simulink model "Two_Level_SVM_No_PV_No_Control_Sw_Benchmark_v2"  (R2022b)
settings: Solver=FixedStepAuto  StartTime=0.0  StopTime=5  FixedStep=1e-7  RelTol=1e-3
model workspace (MAT data in the model file):
  Phase_Shift = Simulink.Parameter
  Phase_Shift.Value = 0.1974
  Phase_Shift.DataType = 'auto'
  Phase_Shift.Complexity = 'real'
  Phase_Shift.Dimensions = [1 1]
  Vrms_p = Simulink.Parameter
  Vrms_p.Value = 285.7229
  Vrms_p.DataType = 'auto'
  Vrms_p.Complexity = 'real'
  Vrms_p.Dimensions = [1 1]
libraries: spsIGBTDiodeLib x6, slpidlib x5, spsThreePhaseVIMeasurementLib x5, spsThreePhaseSeriesRLCBranchLib x4, spsGroundLib x2, spsabctodq0Lib x2, spsdq0toabcLib x1, spsDCVoltageSourceLib x1, spsThreePhaseProgrammableVoltageSourceLib x1, eeGeneralControl x1, spsabctoAlphaBetaZeroLib x1, eePwmGeneratorTwoLevel x1
(part 1 of 2)
settings Model: Creator=nitukeee  LastModifiedBy=buckb
settings OptimizationCC: LifeSpan=inf
settings DebuggingCC: SolverPrmCheckMsg=warning  UnconnectedInputMsg=warning  UnconnectedOutputMsg=warning  UnconnectedLineMsg=warning  SFUnexpectedBacktrackingDiag=warning  SFNoUnconditionalDefaultTransitionDiag=warning  SFExecutionAtInitializationDiag=none  SFMachineParentedDataDiag=warning  ArithmeticOperatorsInVariantConditions=warning
settings HardwareCC: ProdBitPerPointer=32  ProdBitPerSizeT=32  ProdBitPerPtrDiffT=32  ProdLargestAtomicFloat=None  ProdIntDivRoundTo=Undefined  ProdEndianess=Unspecified  ProdWordSize=32  ProdHWDeviceType=32-bit Generic
settings ModelReferenceCC: EnableRefExpFcnMdlSchedulingChecks=on  PropagateSignalLabelsOutOfModel=off
settings SFSimCC: SimUseLocalCustomCode=off  CustomCodeUndefinedFunction=UseInterfaceOnly
settings RTWCC: RTWUseLocalCustomCode=off  DLArmComputeVersion=19.05
settings CodeAppCC: StateflowObjectComments=on
settings GRTTargetCC: TargetLangStandard=C89/C90 (ANSI)
settings ConfigComp: CovMetricSettings=dw  CovSaveCumulativeToWorkspaceVar=on  CovSaveSingleToWorkspaceVar=on  CovExternalEMLEnable=off  CovSFcnEnable=off
settings SimscapeCC: SimscapeNormalizeSystem=off

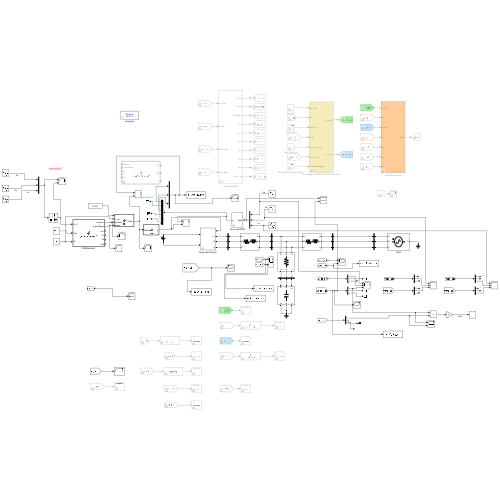
[thumbnail: Simulink's stored preview of the top-level diagram]
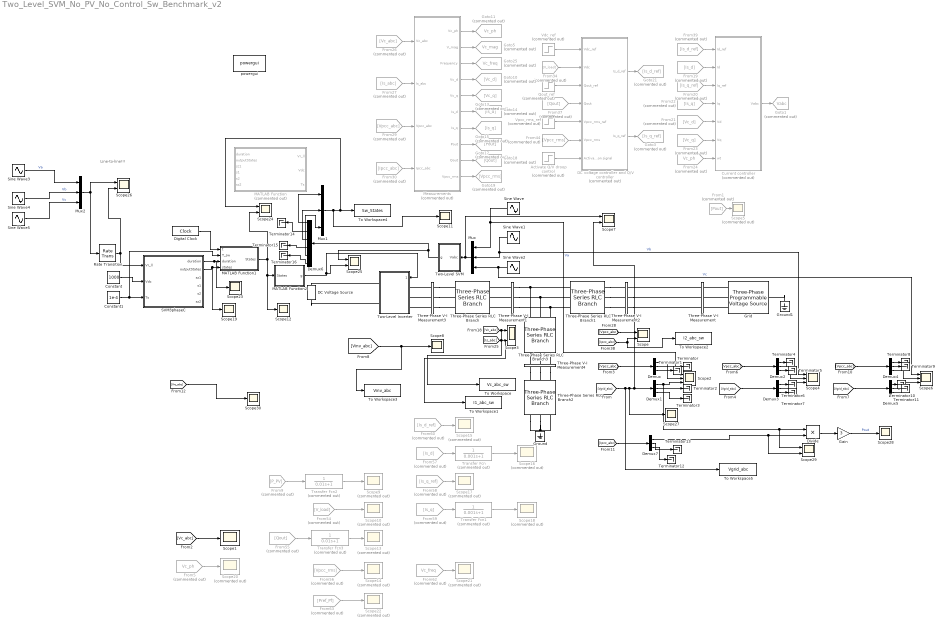
== system Two_Level_SVM_No_PV_No_Control_Sw_Benchmark_v2 ==
  note: Line-to-line!!!
  Activate Q/V droop control : Step  Commented=on  Time=3  After=0  SampleTime=0
  Constant : Constant  Value=1000
  Constant1 : Constant  Value=1e-4
  Current controller : Subsystem  Commented=on  mask{Kp_current_loop=0.59, Ki_current_loop=30, L1=3e-3, Udc_ref=1000, fsw=10e3}
      mask prompts: Kp_current_loop "Proportional parameter of current loop"; Ki_current_loop "Integral parameter of current loop"; L1 "Inverter-side inductor value [H]"; Udc_ref "DC voltage reference [V]"; fsw "Inverter switching frequency [Hz]"
      mask TypeOptions Kp_current_loop: Discrete PID Controller/P | Discrete PID Controller1/P
      mask TypeOptions Ki_current_loop: Discrete PID Controller/I | Discrete PID Controller1/I
      mask TypeOptions L1: L/Gain | L1/Gain
      mask TypeOptions Udc_ref: DC voltage/Value
      mask TypeOptions fsw:
      | PWM Generator
      | (Three-phase, Two-level)/fsw
  DC Voltage Source : spsDCVoltageSourceLib/DC Voltage Source  Amplitude=1000  Measurements=None
  DC voltage controller and Q/V controller : Subsystem  Commented=on  mask(DC voltage controller and Q/V controller){Kp_vdc_control=0.05, Ki_vdc_control=10, Kp_QV_control=1e-3, Ki_QV_control=1e-2, Dq=4.1667e+03}
      mask prompts: Kp_vdc_control "Proportional parameter of DC voltage controller"; Ki_vdc_control "Integratal parameter of DC voltage controller"; Kp_QV_control "Proportional parameter of Q/V controller"; Ki_QV_control "Integral parameter of Q/V controller"; Dq "Q/V droop constant [Var/V]"
      mask TypeOptions Kp_vdc_control: Discrete PID Controller/P
      mask TypeOptions Ki_vdc_control: Discrete PID Controller/I
      mask TypeOptions Kp_QV_control: Discrete PID Controller3/P
      mask TypeOptions Ki_QV_control: Discrete PID Controller3/I
      mask TypeOptions Dq: Dq/Gain
      mask DialogControl ParameterGroupVar1 Prompt: DC voltage controller
      mask DialogControl ParameterGroupVar2 Prompt: Q/V controller
  Demux{,1..5,7} (7 alike) : Demux  Outputs=3
  Demux6 : Demux  Outputs=6
  Digital Clock : DigitalClock  SampleTime=1e-7
  Divide : Product  Inputs=**
  From1 : From  Commented=on  GotoTag=Pout
  From19 : From  Commented=on  GotoTag=Is_d
  From20 : From  Commented=on  GotoTag=Is_q_ref
  From21 : From  Commented=on  GotoTag=Vc_d
  From22 : From  Commented=on  GotoTag=Is_q
  From23 : From  Commented=on  GotoTag=Vc_q
  From24 : From  Commented=on  GotoTag=Vc_ph  TagVisibility=global
  From26 : From  Commented=on  GotoTag=Vc_abc  TagVisibility=global
  From27 : From  Commented=on  GotoTag=Is_abc  TagVisibility=global
  From29 : From  Commented=on  GotoTag=Vpcc_abc  TagVisibility=global
  From30 : From  Commented=on  GotoTag=Ipcc_abc  TagVisibility=global
  From34 : From  Commented=on  GotoTag=V_load
  From37 : From  Commented=on  GotoTag=Qout
  From39 : From  Commented=on  GotoTag=Is_d_ref
  From44 : From  Commented=on  GotoTag=Vpcc_rms
  From5 : From  Commented=on  GotoTag=Vc_ph
  From54 : From  Commented=on  GotoTag=V_load
  From55 : From  Commented=on  GotoTag=Qout
  From56 : From  Commented=on  GotoTag=Vpcc_rms
  From57 : From  Commented=on  GotoTag=Is_d
  From58 : From  Commented=on  GotoTag=Is_q_ref
  From59 : From  Commented=on  GotoTag=Is_q
  From60 : From  Commented=on  GotoTag=Is_d_ref
  From62 : From  Commented=on  GotoTag=Vc_freq  TagVisibility=global
  From63 : From  Commented=on  GotoTag=Pref_Pf
  From9 : From  Commented=on  GotoTag=P_PV
  Gain : Gain  Gain=3
  Goto1 : Goto  Commented=on  GotoTag=Vabc  TagVisibility=global
  Goto10 : Goto  Commented=on  GotoTag=Vc_d
  Goto11 : Goto  Commented=on  GotoTag=Vc_ph  TagVisibility=global
  Goto13 : Goto  Commented=on  GotoTag=Vc_q
  Goto14 : Goto  Commented=on  GotoTag=Is_d
  Goto15 : Goto  Commented=on  GotoTag=Is_q
  Goto17 : Goto  Commented=on  GotoTag=Pout
  Goto18 : Goto  Commented=on  GotoTag=Qout
  Goto19 : Goto  Commented=on  GotoTag=Vpcc_rms
  Goto21 : Goto  Commented=on  GotoTag=Is_d_ref
  Goto25 : Goto  Commented=on  GotoTag=Vc_freq  TagVisibility=global
  Goto3 : Goto  Commented=on  GotoTag=Is_q_ref
  Goto5 : Goto  Commented=on  GotoTag=Vc_mag  TagVisibility=global
  Grid : spsThreePhaseProgrammableVoltageSourceLib/Three-Phase Programmable Voltage Source  PositiveSequence="[480  0 60]"  VariationEntity=None  VariationType=Table of time-amplitude pairs  VariationTypeAlt=Step  VariationStep=-0.1  VariationRate=10  VariationMagnitude=0.3  VariationFrequency=2  VariationTiming=[5.5 6.5]  VariationPhaseA=off  Amplitudes=[1 0.96 1.02]  TimeValues=[0 7 8.5]  HarmonicGeneration=off  HarmonicA=[3 0.2 -25 0]  HarmonicB=[2 0.15 35 2]  Timing="[0.05  3]"  BusType=swing  Pref=0  Qref=0  Qmin=-inf  Qmax=inf
  Ground : spsGroundLib/Ground  LConnTagsString=a
  Ground1 : spsGroundLib/Ground  LConnTagsString=a
  MATLAB Function : MATLAB Function  Commented=on  TreatAsAtomicUnit=on
  MATLAB Function1 : MATLAB Function  TreatAsAtomicUnit=on
  MATLAB Function2 : MATLAB Function  TreatAsAtomicUnit=on
  Measurements : Subsystem  Commented=on  mask{Kp_PLL=100, Ki_PLL=1e5}
      mask prompts: Kp_PLL "Proportional parameter of PLL"; Ki_PLL "Integral parameter of PLL"
      mask TypeOptions Kp_PLL: Phase Locked Loop (PLL)/Discrete PID Controller/P
      mask TypeOptions Ki_PLL: Phase Locked Loop (PLL)/Discrete PID Controller/I
  Mux : Mux  Inputs=3
  Mux1 : Mux  Inputs=3
  Mux2 : Mux  Inputs=3
  Qout_ref : Step  Commented=on  Time=0  After=0  SampleTime=0
  Rate Transition : RateTransition  OutPortSampleTime=1e-4
  SVM3phaseC : MATLAB Function  TreatAsAtomicUnit=on
  Scope{,3,7,24..26,29} (7 alike) : Scope  NumInputPorts=2
  Scope{1,8,11..12,19,23,27..28,30} (9 alike) : Scope
  Scope{5,9..10,13..18,20..22} (12 alike) : Scope  Commented=on
  Scope2 : Scope  NumInputPorts=3
  Scope4 : Scope  NumInputPorts=3
  Scope6 : Scope  NumInputPorts=3
  Sine Wave : Sin  Amplitude=Vrms_p*sqrt(2)  Frequency=2*pi*60  Phase=Phase_Shift  SampleTime=0
  Sine Wave1 : Sin  Amplitude=Vrms_p*sqrt(2)  Frequency=2*pi*60  Phase=4*pi/3+Phase_Shift  SampleTime=0
  Sine Wave2 : Sin  Amplitude=Vrms_p*sqrt(2)  Frequency=2*pi*60  Phase=2*pi/3+Phase_Shift  SampleTime=0
  Sine Wave3 : Sin  Amplitude=Vrms_p*sqrt(2)*sqrt(3)  Frequency=2*pi*60  Phase=Phase_Shift+pi/6+0.02  SampleTime=0
  Sine Wave4 : Sin  Amplitude=Vrms_p*sqrt(2)*sqrt(3)  Frequency=2*pi*60  Phase=4*pi/3+Phase_Shift+pi/6+0.02  SampleTime=0
  Sine Wave5 : Sin  Amplitude=Vrms_p*sqrt(2)*sqrt(3)  Frequency=2*pi*60  Phase=2*pi/3+Phase_Shift+pi/6+0.02  SampleTime=0
  Terminator{,1..16} (17 alike) : Terminator
  Three-Phase Series RLC Branch : spsThreePhaseSeriesRLCBranchLib/Three-Phase Series RLC Branch  LConnTagsString=A|B|C  RConnTagsString=A|B|C  BranchType=RL  Resistance=0.03  Inductance=3e-4  Capacitance=1e-6  Measurements=None
  Three-Phase Series RLC Branch1 : spsThreePhaseSeriesRLCBranchLib/Three-Phase Series RLC Branch  LConnTagsString=A|B|C  RConnTagsString=A|B|C  BranchType=RL  Resistance=0.0053  Inductance=9.3183e-4  Capacitance=1e-6  Measurements=None
  Three-Phase Series RLC Branch2 : spsThreePhaseSeriesRLCBranchLib/Three-Phase Series RLC Branch  LConnTagsString=A|B|C  RConnTagsString=A|B|C  BranchType=C  Resistance=1  Inductance=1e-3  Capacitance=9.7860e-5  Measurements=None
  Three-Phase Series RLC Branch3 : spsThreePhaseSeriesRLCBranchLib/Three-Phase Series RLC Branch  LConnTagsString=A|B|C  RConnTagsString=A|B|C  BranchType=R  Resistance=1  Inductance=1e-3  Capacitance=9.7860e-5  Measurements=None
  Three-Phase V-I Measurement : spsThreePhaseVIMeasurementLib/Three-Phase V-I Measurement  VoltageMeasurement=phase-to-ground  SetLabelV=on  LabelV=Vgrid_abc  Vpu=off  VpuLL=off  CurrentMeasurement=yes  SetLabelI=on  LabelI=Igrid_abc  Ipu=off  Pbase=100e6  Vbase=500e3  OutputType=Complex  PhasorSimulation=off  PSBequivalent=0
  Three-Phase V-I Measurement1 : spsThreePhaseVIMeasurementLib/Three-Phase V-I Measurement  VoltageMeasurement=phase-to-ground  SetLabelV=on  LabelV=Vrc_abc  Vpu=off  VpuLL=off  CurrentMeasurement=yes  SetLabelI=on  LabelI=Is_abc  Ipu=off  Pbase=100e6  Vbase=500e3  OutputType=Complex  PhasorSimulation=off  PSBequivalent=0
  Three-Phase V-I Measurement2 : spsThreePhaseVIMeasurementLib/Three-Phase V-I Measurement  VoltageMeasurement=phase-to-ground  SetLabelV=on  LabelV=Vpcc_abc  Vpu=off  VpuLL=off  CurrentMeasurement=yes  SetLabelI=on  LabelI=Ipcc_abc  Ipu=off  Pbase=100e6  Vbase=500e3  OutputType=Complex  PhasorSimulation=off  PSBequivalent=0
  Three-Phase V-I Measurement3 : spsThreePhaseVIMeasurementLib/Three-Phase V-I Measurement  VoltageMeasurement=phase-to-ground  SetLabelV=on  LabelV=Vinv_abc  Vpu=off  VpuLL=off  CurrentMeasurement=yes  SetLabelI=on  LabelI=Is_abc_2  Ipu=off  Pbase=100e6  Vbase=500e3  OutputType=Complex  PhasorSimulation=off  PSBequivalent=0
  Three-Phase V-I Measurement4 : spsThreePhaseVIMeasurementLib/Three-Phase V-I Measurement  VoltageMeasurement=phase-to-ground  SetLabelV=on  LabelV=Vc_abc  Vpu=off  VpuLL=off  CurrentMeasurement=yes  SetLabelI=on  LabelI=Ic_abc  Ipu=off  Pbase=100e6  Vbase=500e3  OutputType=Complex  PhasorSimulation=off  PSBequivalent=0
  To Workspace : ToWorkspace  VariableName=Vc_abc_sw  SaveFormat=Timeseries  SampleTime=-1
  To Workspace1 : ToWorkspace  VariableName=I1_abc_sw  SaveFormat=Timeseries  SampleTime=-1
  To Workspace2 : ToWorkspace  VariableName=I2_abc_sw  SaveFormat=Timeseries  SampleTime=-1
  To Workspace3 : ToWorkspace  VariableName=Vinv_abc  SaveFormat=Timeseries  SampleTime=-1
  To Workspace4 : ToWorkspace  VariableName=Sw_States  SaveFormat=Timeseries  SampleTime=-1
  To Workspace5 : ToWorkspace  VariableName=Vgrid_abc  SaveFormat=Timeseries  SampleTime=-1
  Transfer Fcn : TransferFcn  Commented=on  Denominator=[0.001 1]
  Transfer Fcn1 : TransferFcn  Commented=on  Denominator=[0.001 1]
  Transfer Fcn2 : TransferFcn  Commented=on  Denominator=[0.01 1]
  Transfer Fcn3 : TransferFcn  Commented=on  Denominator=[0.01 1]
  Two-Level Inverter : Subsystem  mask{Ron=0.2e-5, Rs=5e8, Cs=inf, CDC=10351e-6}
      mask prompts: Ron "Device On-State Resistance [Ohms]"; Rs "Snubber Resistance [Ohms]"; Cs "Snubber Capacitance [F]"; CDC "DC-Link Capacitance [F]"
      mask DialogControl DescGroupVar Prompt: Two-Level Inverter
      mask DialogControl DescTextVar Prompt: Two-level inverter model that makes use of IGBT discrete devices
  Two-Level SVM : Subsystem  mask{Udc_ref=1000, fsw=10e3}
      mask prompts: Udc_ref "DC Voltage Reference [V]"; fsw "Inverter Switching Frequency [Hz]"
      mask DialogControl DescGroupVar Prompt: Two-Level SVM
      mask DialogControl DescTextVar Prompt: Standard SVM scheme for a two-level inverter
  Vdc_ref : Step  Commented=on  Time=0.5  Before=1000  After=1000  SampleTime=0
  Vpcc_rms_ref : Step  Commented=on  Time=0.5  Before=480  After=480  SampleTime=0
  powergui : spspowerguiLib/powergui  Priority=1  SimulationMode=Discrete  SampleTime=1e-7  frequency=60  Iterations=50  frequencyindice=0  Pbase=100e6  ErrMax=1e-4  UnitsV=kV  UnitsW=MW  buscounter=0  FunctionMessages=off  echomessages=off  EnableUseOfTLC=off  CurrentSourceSwitches=off  DisableSnubberDevices=off  DisableRonSwitches=off  DisableVfSwitches=off  DisplayEquations=off  AutomaticDiscreteSolvers=off  SolverType=Tustin/Backward Euler (TBE)  Interpol=off  ExternalGateDelay=off  methode=off  Ts=100  x0status=blocks  SPID=on  SwTol=0  HookPort=off  NonlinearTolerance=1e-4  nMaxIteration=100  ContinueOnMaxIteration=off  RestoreLinks=warning  ResistiveCurrentMeasurement=off  Frange=[0:2:500]  Ylog=off  Xlog=on  ShowGrid=off  save=off  variable=ZData  structure=0  ZoomFFT=off  StartTime=0.0  cycles=1  DisplayStyle=1  fundamental=60  FreqAxis=off  MaxFrequency=1000  frequencyindicesteady=1  RmsSteady=1  display=off
  wires:
  From21/1 -> Current controller/5(Vd)
  From39/1 -> Current controller/1(Id_ref)
  From19/1 -> Current controller/2(Id)
  From22/1 -> Current controller/4(Iq)
  From23/1 -> Current controller/6(Vq)
  From24/1 -> Current controller/7(wt)
  Current controller/1(Vabc) -> Goto1/1
  From20/1 -> Current controller/3(Iq_ref)
  Vdc_ref/1 -> DC voltage controller and Q/V controller/1(Vdc_ref)
  From34/1 -> DC voltage controller and Q/V controller/2(Vdc)
  Qout_ref/1 -> DC voltage controller and Q/V controller/3(Qout_ref)
  From37/1 -> DC voltage controller and Q/V controller/4(Qout)
  Vpcc_rms_ref/1 -> DC voltage controller and Q/V controller/5(Vpcc_rms_ref)
  From44/1 -> DC voltage controller and Q/V controller/6(Vpcc_rms)
  Activate Q/V droop control/1 -> DC voltage controller and Q/V controller/7(Activation signal)
  DC voltage controller and Q/V controller/1(Is_d_ref) -> Goto21/1
  DC voltage controller and Q/V controller/2(Is_q_ref) -> Goto3/1
  From26/1 -> Measurements/1(Vc_abc)
  From27/1 -> Measurements/2(Is_abc)
  From29/1 -> Measurements/3(Vpcc_abc)
  Measurements/1(Vc_ph) -> Goto11/1
  Measurements/2(V_mag) -> Goto5/1
  Measurements/3(Frequency) -> Goto25/1
  Measurements/4(Vc_d) -> Goto10/1
  Measurements/5(Vc_q) -> Goto13/1
  Measurements/6(Is_d) -> Goto14/1
  Measurements/8(Pout) -> Goto17/1
  Measurements/9(Qout) -> Goto18/1
  Measurements/10(Vpcc_rms) -> Goto19/1
  Measurements/7(Is_q) -> Goto15/1
  From30/1 -> Measurements/4(Ipcc_abc)
  From9/1 -> Transfer Fcn2/1
  From54/1 -> Scope10/1
  From55/1 -> Transfer Fcn3/1
  From56/1 -> Scope14/1
  From58/1 -> Scope17/1
  From57/1 -> Transfer Fcn/1
  From59/1 -> Transfer Fcn1/1
  From60/1 -> Scope15/1
  Transfer Fcn/1 -> Scope16/1
  Transfer Fcn1/1 -> Scope18/1
  Transfer Fcn2/1 -> Scope9/1
  [Vc_abc] -> Scope1/1
  From5/1 -> Scope20/1
  From62/1 -> Scope21/1
  Transfer Fcn3/1 -> Scope13/1
  From63/1 -> Scope22/1
  Two-Level SVM/1(g) -> Scope25/1, Demux6/1
  [Is_abc] -> To Workspace1/1, Scope3/2
  [Vc_abc] -> To Workspace/1, Scope3/1
  [Vpcc_abc] -> Scope/1
  [Ipcc_abc] -> To Workspace2/1, Scope/2
  From1/1 -> Scope5/1
  [Vinv_abc] -> Scope8/1, To Workspace3/1
  Mux/1 -> Scope7/1, Two-Level SVM/1(Vabc)
  Sine Wave/1 -> Scope2/1, Mux/1  "Va"
  Sine Wave1/1 -> Scope4/1, Mux/2  "Vb"
  Sine Wave2/1 -> Scope6/1, Mux/3  "Vc"
  [Vpcc_abc] -> Demux/1
  Demux/1 -> Scope2/2
  [Vgrid_abc] -> To Workspace5/1, Scope27/1, Scope7/2, Demux1/1
  Demux1/1 -> Scope29/1, Divide/1, Scope2/3
  [Vgrid_abc] -> Demux3/1
  [Vpcc_abc] -> Demux2/1
  Demux2/2 -> Scope4/2
  Demux3/2 -> Scope4/3
  [Vpcc_abc] -> Demux4/1
  [Vgrid_abc] -> Demux5/1
  Demux4/3 -> Scope6/2
  Demux5/3 -> Scope6/3
  Demux/2 -> Terminator/1
  Demux/3 -> Terminator1/1
  Demux1/2 -> Terminator2/1
  Demux1/3 -> Terminator3/1
  Demux2/1 -> Terminator4/1
  Demux2/3 -> Terminator5/1
  Demux3/1 -> Terminator6/1
  Demux3/3 -> Terminator7/1
  Demux4/1 -> Terminator8/1
  Demux4/2 -> Terminator9/1
  Demux5/1 -> Terminator10/1
  Demux5/2 -> Terminator11/1
  Mux1/1 -> Scope11/1, Scope24/1, To Workspace4/1
  Demux6/1 -> Mux1/1
  Demux6/3 -> Mux1/2
  Demux6/5 -> Mux1/3
  Constant/1 -> SVM3phaseC/2(Vdc)
  Constant1/1 -> MATLAB Function1/2(T_sw), SVM3phaseC/3(Ts)
  Rate Transition/1 -> SVM3phaseC/1(Vr_ll), Scope26/2
  Digital Clock/1 -> MATLAB Function1/1(t)
  SVM3phaseC/1(duration) -> Scope23/1, MATLAB Function1/3(duration)
  SVM3phaseC/2(outputStates) -> Scope19/1, MATLAB Function1/4(states)
  MATLAB Function1/1(States) -> MATLAB Function2/1(States), Scope12/1, Scope24/2
  Mux2/1 -> Rate Transition/1, Scope26/1
  Sine Wave3/1 -> Mux2/1  "Va"
  Sine Wave5/1 -> Mux2/3  "Vc"
  Sine Wave4/1 -> Mux2/2  "Vb"
  MATLAB Function2/1(g) -> Two-Level Inverter/1("  "), Scope25/2
  [Ipcc_abc] -> Demux7/1
  Demux7/1 -> Scope29/2, Divide/2
  Demux7/3 -> Terminator12/1
  Demux7/2 -> Terminator13/1
  Divide/1 -> Gain/1
  Gain/1 -> Scope28/1  "Pout"
  [Vrc_abc] -> Scope30/1
  Demux6/2 -> Terminator14/1
  Demux6/4 -> Terminator15/1
  Demux6/6 -> Terminator16/1
  connections:
  Three-Phase V-I Measurement1/RConn1 -- Three-Phase Series RLC Branch3/LConn1 -- Three-Phase Series RLC Branch1/LConn1
  Three-Phase V-I Measurement1/RConn2 -- Three-Phase Series RLC Branch3/LConn2 -- Three-Phase Series RLC Branch1/LConn2
  Three-Phase V-I Measurement1/RConn3 -- Three-Phase Series RLC Branch3/LConn3 -- Three-Phase Series RLC Branch1/LConn3
  Three-Phase Series RLC Branch2/RConn1 -- Three-Phase Series RLC Branch2/RConn2 -- Ground/LConn1 -- Three-Phase Series RLC Branch2/RConn3
  Three-Phase V-I Measurement1/LConn1 -- Three-Phase Series RLC Branch/RConn1
  Three-Phase V-I Measurement1/LConn2 -- Three-Phase Series RLC Branch/RConn2
  Three-Phase V-I Measurement1/LConn3 -- Three-Phase Series RLC Branch/RConn3
  Grid/RConn1 -- Three-Phase V-I Measurement/RConn1
  Grid/RConn2 -- Three-Phase V-I Measurement/RConn2
  Grid/RConn3 -- Three-Phase V-I Measurement/RConn3
  Three-Phase Series RLC Branch1/RConn1 -- Three-Phase V-I Measurement2/LConn1
  Three-Phase Series RLC Branch1/RConn2 -- Three-Phase V-I Measurement2/LConn2
  Three-Phase Series RLC Branch1/RConn3 -- Three-Phase V-I Measurement2/LConn3
  Three-Phase V-I Measurement3/RConn1 -- Three-Phase Series RLC Branch/LConn1
  Three-Phase V-I Measurement3/RConn2 -- Three-Phase Series RLC Branch/LConn2
  Three-Phase V-I Measurement3/RConn3 -- Three-Phase Series RLC Branch/LConn3
  Three-Phase V-I Measurement3/LConn3 -- Two-Level Inverter/LConn3
  Three-Phase V-I Measurement3/LConn2 -- Two-Level Inverter/LConn2
  Three-Phase V-I Measurement3/LConn1 -- Two-Level Inverter/LConn1
  DC Voltage Source/LConn1 -- Two-Level Inverter/RConn2
  Two-Level Inverter/RConn1 -- DC Voltage Source/RConn1
  Ground1/LConn1 -- Grid/LConn1
  Three-Phase V-I Measurement2/RConn2 -- Three-Phase V-I Measurement/LConn2
  Three-Phase V-I Measurement2/RConn3 -- Three-Phase V-I Measurement/LConn3
  Three-Phase V-I Measurement/LConn1 -- Three-Phase V-I Measurement2/RConn1
  Three-Phase V-I Measurement4/LConn1 -- Three-Phase Series RLC Branch3/RConn1
  Three-Phase V-I Measurement4/LConn2 -- Three-Phase Series RLC Branch3/RConn2
  Three-Phase V-I Measurement4/LConn3 -- Three-Phase Series RLC Branch3/RConn3
  Three-Phase V-I Measurement4/RConn1 -- Three-Phase Series RLC Branch2/LConn1
  Three-Phase V-I Measurement4/RConn2 -- Three-Phase Series RLC Branch2/LConn2
  Three-Phase V-I Measurement4/RConn3 -- Three-Phase Series RLC Branch2/LConn3

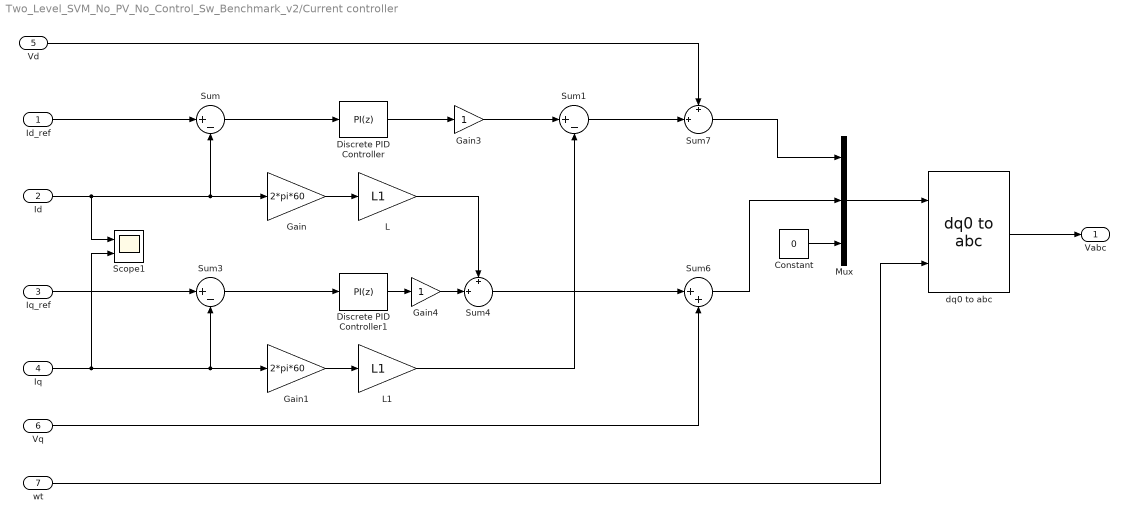
== system Two_Level_SVM_No_PV_No_Control_Sw_Benchmark_v2/Current controller ==
  Id_ref : Inport
  Id : Inport  Port=2
  Iq_ref : Inport  Port=3
  Iq : Inport  Port=4
  Vd : Inport  Port=5
  Vq : Inport  Port=6
  wt : Inport  Port=7
  Constant : Constant  Value=0
  Discrete PID Controller : slpidlib/PID Controller  Controller=PI  Form=Parallel  TimeDomain=Discrete-time  UseExternalTs=off  SampleTime=-1  IntegratorMethod=Forward Euler  FilterMethod=Forward Euler  ControllerParametersSource=internal  P=Kp_current_loop  I=Ki_current_loop  UseKiTs=off  D=0  N=100  UseFilter=on  TunerSelectOption=Transfer Function Based (PID Tuner App)  InitialConditionSource=internal  InitialConditionForIntegrator=0  InitialConditionForFilter=0  DifferentiatorICPrevScaledInput=0  ExternalReset=none  TrackingMode=off  Kt=1  LimitOutput=off  SatLimitsSource=internal  UpperSaturationLimit=inf  LowerSaturationLimit=-inf  LinearizeAsGain=off  AntiWindupMode=none  Kb=1  LimitIntegrator=off  UpperIntegratorSaturationLimit=inf  LowerIntegratorSaturationLimit=-inf  POutMin=[]  POutMax=[]  IOutMin=[]  IOutMax=[]  DOutMin=[]  DOutMax=[]  NOutMin=[]  NOutMax=[]  SumOutMin=[]  SumOutMax=[]  SaturationOutMin=[]  SaturationOutMax=[]  PParamMin=[]  PParamMax=[]  IParamMin=[]  IParamMax=[]  DParamMin=[]  DParamMax=[]  NParamMin=[]  NParamMax=[]  KbParamMin=[]  KbParamMax=[]  KtParamMin=[]  KtParamMax=[]  KbOutMin=[]  KbOutMax=[]  KtOutMin=[]  KtOutMax=[]  IntegratorOutMin=[]  IntegratorOutMax=[]  FilterOutMin=[]  FilterOutMax=[]  SumI1OutMin=[]  SumI1OutMax=[]  SumI2OutMin=[]  SumI2OutMax=[]  SumI3OutMin=[]  SumI3OutMax=[]  SumI4OutMin=[]  SumI4OutMax=[]  SumDOutMin=[]  SumDOutMax=[]  DifferentiatorOutMin=[]  DifferentiatorOutMax=[]  FilterDiffOutCoefMin=[]  FilterDiffOutCoefMax=[]  ReciprocalOutMin=[]  ReciprocalOutMax=[]  SumDenOutMin=[]  SumDenOutMax=[]  SumNumOutMin=[]  SumNumOutMax=[]  DivideOutMin=[]  DivideOutMax=[]  UdiffTsProdOutMin=[]  UdiffTsProdOutMax=[]  NTsProdOutMin=[]  NTsProdOutMax=[]  UintegralTsProdOutMin=[]  UintegralTsProdOutMax=[]  UngainTsProdOutMin=[]  UngainTsProdOutMax=[]  ClampingZeroOutDataTypeStr=Inherit: Inherit via back propagation  ClampingZeroOutMin=[]  ClampingZeroOutMax=[]  FilterDenConstantOutDataTypeStr=Inherit: Inherit via back propagation  FilterDenConstantOutMin=[]  FilterDenConstantOutMax=[]  PCopyOutDataTypeStr=Inherit: Inherit via back propagation  PCopyOutMin=[]  PCopyOutMax=[]  NCopyOutDataTypeStr=Inherit: Inherit via back propagation  NCopyOutMin=[]  NCopyOutMax=[]  IntegratorContinuousStateAttributes=''  IntegratorStateMustResolveToSignalObject=off  IntegratorRTWStateStorageClass=Auto  FilterContinuousStateAttributes=''  FilterStateMustResolveToSignalObject=off  FilterRTWStateStorageClass=Auto  ParallelPVariant=InternalParameters  IdealPVariant=Disabled  IVariant=InternalParameters  DVariant=Disabled  IntegratorVariant=Discrete  SatVariant=Disabled  AWVariant=Passthrough  PCopyVariant=Disabled  TRVariant=Disabled  FdbkBlocksVariant=Forward  IdealPFdbkVariant=Disabled  SatFdbkVariant=Disabled  DerivativeFilterVariant=Disabled  NVariant=Disabled  NCopyVariant=Disabled_SignalSpec  FilterICVariant=Disabled  IntegratorICVariant=InternalICs  ExternalResetVariant=Disabled  TRSumVariant=Passthrough  SumFdbkVariant=Disabled  SumVariant=Sum_PI  TsampFilterVariant=InternalTs  TsampNgainVariant=Passthrough  TsampIntegralVariant=Passthrough  ExternalSaturationOutDataTypeStr=Inherit: Same as second input
  Discrete PID Controller1 : slpidlib/PID Controller  Controller=PI  Form=Parallel  TimeDomain=Discrete-time  UseExternalTs=off  SampleTime=-1  IntegratorMethod=Forward Euler  FilterMethod=Forward Euler  ControllerParametersSource=internal  P=Kp_current_loop  I=Ki_current_loop  UseKiTs=off  D=0  N=100  UseFilter=on  TunerSelectOption=Transfer Function Based (PID Tuner App)  InitialConditionSource=internal  InitialConditionForIntegrator=0  InitialConditionForFilter=0  DifferentiatorICPrevScaledInput=0  ExternalReset=none  TrackingMode=off  Kt=1  LimitOutput=off  SatLimitsSource=internal  UpperSaturationLimit=inf  LowerSaturationLimit=-inf  LinearizeAsGain=off  AntiWindupMode=none  Kb=1  LimitIntegrator=off  UpperIntegratorSaturationLimit=inf  LowerIntegratorSaturationLimit=-inf  POutMin=[]  POutMax=[]  IOutMin=[]  IOutMax=[]  DOutMin=[]  DOutMax=[]  NOutMin=[]  NOutMax=[]  SumOutMin=[]  SumOutMax=[]  SaturationOutMin=[]  SaturationOutMax=[]  PParamMin=[]  PParamMax=[]  IParamMin=[]  IParamMax=[]  DParamMin=[]  DParamMax=[]  NParamMin=[]  NParamMax=[]  KbParamMin=[]  KbParamMax=[]  KtParamMin=[]  KtParamMax=[]  KbOutMin=[]  KbOutMax=[]  KtOutMin=[]  KtOutMax=[]  IntegratorOutMin=[]  IntegratorOutMax=[]  FilterOutMin=[]  FilterOutMax=[]  SumI1OutMin=[]  SumI1OutMax=[]  SumI2OutMin=[]  SumI2OutMax=[]  SumI3OutMin=[]  SumI3OutMax=[]  SumI4OutMin=[]  SumI4OutMax=[]  SumDOutMin=[]  SumDOutMax=[]  DifferentiatorOutMin=[]  DifferentiatorOutMax=[]  FilterDiffOutCoefMin=[]  FilterDiffOutCoefMax=[]  ReciprocalOutMin=[]  ReciprocalOutMax=[]  SumDenOutMin=[]  SumDenOutMax=[]  SumNumOutMin=[]  SumNumOutMax=[]  DivideOutMin=[]  DivideOutMax=[]  UdiffTsProdOutMin=[]  UdiffTsProdOutMax=[]  NTsProdOutMin=[]  NTsProdOutMax=[]  UintegralTsProdOutMin=[]  UintegralTsProdOutMax=[]  UngainTsProdOutMin=[]  UngainTsProdOutMax=[]  ClampingZeroOutDataTypeStr=Inherit: Inherit via back propagation  ClampingZeroOutMin=[]  ClampingZeroOutMax=[]  FilterDenConstantOutDataTypeStr=Inherit: Inherit via back propagation  FilterDenConstantOutMin=[]  FilterDenConstantOutMax=[]  PCopyOutDataTypeStr=Inherit: Inherit via back propagation  PCopyOutMin=[]  PCopyOutMax=[]  NCopyOutDataTypeStr=Inherit: Inherit via back propagation  NCopyOutMin=[]  NCopyOutMax=[]  IntegratorContinuousStateAttributes=''  IntegratorStateMustResolveToSignalObject=off  IntegratorRTWStateStorageClass=Auto  FilterContinuousStateAttributes=''  FilterStateMustResolveToSignalObject=off  FilterRTWStateStorageClass=Auto  ParallelPVariant=InternalParameters  IdealPVariant=Disabled  IVariant=InternalParameters  DVariant=Disabled  IntegratorVariant=Discrete  SatVariant=Disabled  AWVariant=Passthrough  PCopyVariant=Disabled  TRVariant=Disabled  FdbkBlocksVariant=Forward  IdealPFdbkVariant=Disabled  SatFdbkVariant=Disabled  DerivativeFilterVariant=Disabled  NVariant=Disabled  NCopyVariant=Disabled_SignalSpec  FilterICVariant=Disabled  IntegratorICVariant=InternalICs  ExternalResetVariant=Disabled  TRSumVariant=Passthrough  SumFdbkVariant=Disabled  SumVariant=Sum_PI  TsampFilterVariant=InternalTs  TsampNgainVariant=Passthrough  TsampIntegralVariant=Passthrough  ExternalSaturationOutDataTypeStr=Inherit: Same as second input
  Gain : Gain  Gain=2*pi*60
  Gain1 : Gain  Gain=2*pi*60
  Gain3 : Gain
  Gain4 : Gain
  L : Gain  Gain=L1
  L1 : Gain  Gain=L1
  Mux : Mux  Inputs=3
  Scope1 : Scope  NumInputPorts=2
  Sum : Sum  Inputs=|+-
  Sum1 : Sum  Inputs=|+-
  Sum3 : Sum  Inputs=|+-
  Sum4 : Sum  Inputs=+|+||
  Sum6 : Sum  Inputs=|++
  Sum7 : Sum  Inputs=+|+||
  dq0 to abc : spsdq0toabcLib/dq0 to abc  Alignment=Aligned with phase A axis
  Vabc : Outport
  wires:
  Iq/1 -> Gain1/1, Sum3/2, Scope1/2
  Constant/1 -> Mux/3
  wt/1 -> dq0 to abc/2
  Sum4/1 -> Sum6/1
  Id/1 -> Gain/1, Sum/2, Scope1/1
  Vd/1 -> Sum7/1
  Mux/1 -> dq0 to abc/1
  Discrete PID Controller1/1 -> Gain4/1
  Sum1/1 -> Sum7/2
  Gain/1 -> L/1
  Discrete PID Controller/1 -> Gain3/1
  Sum/1 -> Discrete PID Controller/1
  Sum3/1 -> Discrete PID Controller1/1
  Vq/1 -> Sum6/2
  Gain1/1 -> L1/1
  L/1 -> Sum4/1
  Sum7/1 -> Mux/1
  L1/1 -> Sum1/2
  Sum6/1 -> Mux/2
  Iq_ref/1 -> Sum3/1
  Id_ref/1 -> Sum/1
  Gain3/1 -> Sum1/1
  Gain4/1 -> Sum4/2
  dq0 to abc/1 -> Vabc/1

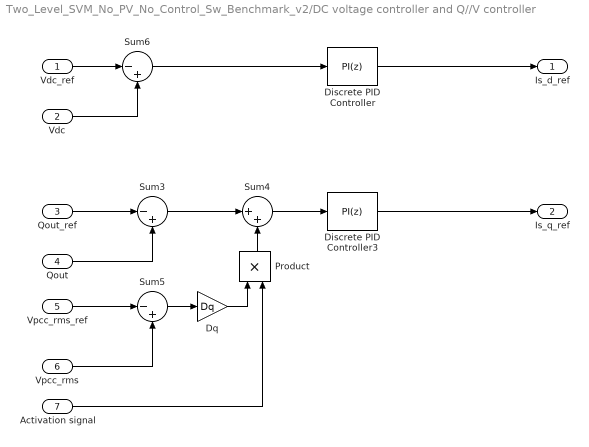
== system Two_Level_SVM_No_PV_No_Control_Sw_Benchmark_v2/DC voltage controller and Q//V controller ==
  Vdc_ref : Inport
  Vdc : Inport  Port=2
  Qout_ref : Inport  Port=3
  Qout : Inport  Port=4
  Vpcc_rms_ref : Inport  Port=5
  Vpcc_rms : Inport  Port=6
  Activation signal : Inport  Port=7
  Discrete PID Controller : slpidlib/PID Controller  Controller=PI  Form=Parallel  TimeDomain=Discrete-time  UseExternalTs=off  SampleTime=-1  IntegratorMethod=Forward Euler  FilterMethod=Forward Euler  ControllerParametersSource=internal  P=Kp_vdc_control  I=Ki_vdc_control  UseKiTs=off  D=0  N=100  UseFilter=on  TunerSelectOption=Transfer Function Based (PID Tuner App)  InitialConditionSource=internal  InitialConditionForIntegrator=0  InitialConditionForFilter=0  DifferentiatorICPrevScaledInput=0  ExternalReset=none  TrackingMode=off  Kt=1  LimitOutput=off  SatLimitsSource=internal  UpperSaturationLimit=inf  LowerSaturationLimit=-inf  LinearizeAsGain=off  AntiWindupMode=none  Kb=1  LimitIntegrator=off  UpperIntegratorSaturationLimit=inf  LowerIntegratorSaturationLimit=-inf  POutMin=[]  POutMax=[]  IOutMin=[]  IOutMax=[]  DOutMin=[]  DOutMax=[]  NOutMin=[]  NOutMax=[]  SumOutMin=[]  SumOutMax=[]  SaturationOutMin=[]  SaturationOutMax=[]  PParamMin=[]  PParamMax=[]  IParamMin=[]  IParamMax=[]  DParamMin=[]  DParamMax=[]  NParamMin=[]  NParamMax=[]  KbParamMin=[]  KbParamMax=[]  KtParamMin=[]  KtParamMax=[]  KbOutMin=[]  KbOutMax=[]  KtOutMin=[]  KtOutMax=[]  IntegratorOutMin=[]  IntegratorOutMax=[]  FilterOutMin=[]  FilterOutMax=[]  SumI1OutMin=[]  SumI1OutMax=[]  SumI2OutMin=[]  SumI2OutMax=[]  SumI3OutMin=[]  SumI3OutMax=[]  SumI4OutMin=[]  SumI4OutMax=[]  SumDOutMin=[]  SumDOutMax=[]  DifferentiatorOutMin=[]  DifferentiatorOutMax=[]  FilterDiffOutCoefMin=[]  FilterDiffOutCoefMax=[]  ReciprocalOutMin=[]  ReciprocalOutMax=[]  SumDenOutMin=[]  SumDenOutMax=[]  SumNumOutMin=[]  SumNumOutMax=[]  DivideOutMin=[]  DivideOutMax=[]  UdiffTsProdOutMin=[]  UdiffTsProdOutMax=[]  NTsProdOutMin=[]  NTsProdOutMax=[]  UintegralTsProdOutMin=[]  UintegralTsProdOutMax=[]  UngainTsProdOutMin=[]  UngainTsProdOutMax=[]  ClampingZeroOutDataTypeStr=Inherit: Inherit via back propagation  ClampingZeroOutMin=[]  ClampingZeroOutMax=[]  FilterDenConstantOutDataTypeStr=Inherit: Inherit via back propagation  FilterDenConstantOutMin=[]  FilterDenConstantOutMax=[]  PCopyOutDataTypeStr=Inherit: Inherit via back propagation  PCopyOutMin=[]  PCopyOutMax=[]  NCopyOutDataTypeStr=Inherit: Inherit via back propagation  NCopyOutMin=[]  NCopyOutMax=[]  IntegratorContinuousStateAttributes=''  IntegratorStateMustResolveToSignalObject=off  IntegratorRTWStateStorageClass=Auto  FilterContinuousStateAttributes=''  FilterStateMustResolveToSignalObject=off  FilterRTWStateStorageClass=Auto  ParallelPVariant=InternalParameters  IdealPVariant=Disabled  IVariant=InternalParameters  DVariant=Disabled  IntegratorVariant=Discrete  SatVariant=Disabled  AWVariant=Passthrough  PCopyVariant=Disabled  TRVariant=Disabled  FdbkBlocksVariant=Forward  IdealPFdbkVariant=Disabled  SatFdbkVariant=Disabled  DerivativeFilterVariant=Disabled  NVariant=Disabled  NCopyVariant=Disabled_SignalSpec  FilterICVariant=Disabled  IntegratorICVariant=InternalICs  ExternalResetVariant=Disabled  TRSumVariant=Passthrough  SumFdbkVariant=Disabled  SumVariant=Sum_PI  TsampFilterVariant=InternalTs  TsampNgainVariant=Passthrough  TsampIntegralVariant=Passthrough  ExternalSaturationOutDataTypeStr=Inherit: Same as second input
  Discrete PID Controller3 : slpidlib/PID Controller  Controller=PI  Form=Parallel  TimeDomain=Discrete-time  UseExternalTs=off  SampleTime=-1  IntegratorMethod=Forward Euler  FilterMethod=Forward Euler  ControllerParametersSource=internal  P=Kp_QV_control  I=Ki_QV_control  UseKiTs=off  D=0  N=100  UseFilter=on  TunerSelectOption=Transfer Function Based (PID Tuner App)  InitialConditionSource=internal  InitialConditionForIntegrator=0  InitialConditionForFilter=0  DifferentiatorICPrevScaledInput=0  ExternalReset=none  TrackingMode=off  Kt=1  LimitOutput=off  SatLimitsSource=internal  UpperSaturationLimit=inf  LowerSaturationLimit=-inf  LinearizeAsGain=off  AntiWindupMode=none  Kb=1  LimitIntegrator=off  UpperIntegratorSaturationLimit=inf  LowerIntegratorSaturationLimit=-inf  POutMin=[]  POutMax=[]  IOutMin=[]  IOutMax=[]  DOutMin=[]  DOutMax=[]  NOutMin=[]  NOutMax=[]  SumOutMin=[]  SumOutMax=[]  SaturationOutMin=[]  SaturationOutMax=[]  PParamMin=[]  PParamMax=[]  IParamMin=[]  IParamMax=[]  DParamMin=[]  DParamMax=[]  NParamMin=[]  NParamMax=[]  KbParamMin=[]  KbParamMax=[]  KtParamMin=[]  KtParamMax=[]  KbOutMin=[]  KbOutMax=[]  KtOutMin=[]  KtOutMax=[]  IntegratorOutMin=[]  IntegratorOutMax=[]  FilterOutMin=[]  FilterOutMax=[]  SumI1OutMin=[]  SumI1OutMax=[]  SumI2OutMin=[]  SumI2OutMax=[]  SumI3OutMin=[]  SumI3OutMax=[]  SumI4OutMin=[]  SumI4OutMax=[]  SumDOutMin=[]  SumDOutMax=[]  DifferentiatorOutMin=[]  DifferentiatorOutMax=[]  FilterDiffOutCoefMin=[]  FilterDiffOutCoefMax=[]  ReciprocalOutMin=[]  ReciprocalOutMax=[]  SumDenOutMin=[]  SumDenOutMax=[]  SumNumOutMin=[]  SumNumOutMax=[]  DivideOutMin=[]  DivideOutMax=[]  UdiffTsProdOutMin=[]  UdiffTsProdOutMax=[]  NTsProdOutMin=[]  NTsProdOutMax=[]  UintegralTsProdOutMin=[]  UintegralTsProdOutMax=[]  UngainTsProdOutMin=[]  UngainTsProdOutMax=[]  ClampingZeroOutDataTypeStr=Inherit: Inherit via back propagation  ClampingZeroOutMin=[]  ClampingZeroOutMax=[]  FilterDenConstantOutDataTypeStr=Inherit: Inherit via back propagation  FilterDenConstantOutMin=[]  FilterDenConstantOutMax=[]  PCopyOutDataTypeStr=Inherit: Inherit via back propagation  PCopyOutMin=[]  PCopyOutMax=[]  NCopyOutDataTypeStr=Inherit: Inherit via back propagation  NCopyOutMin=[]  NCopyOutMax=[]  IntegratorContinuousStateAttributes=''  IntegratorStateMustResolveToSignalObject=off  IntegratorRTWStateStorageClass=Auto  FilterContinuousStateAttributes=''  FilterStateMustResolveToSignalObject=off  FilterRTWStateStorageClass=Auto  ParallelPVariant=InternalParameters  IdealPVariant=Disabled  IVariant=InternalParameters  DVariant=Disabled  IntegratorVariant=Discrete  SatVariant=Disabled  AWVariant=Passthrough  PCopyVariant=Disabled  TRVariant=Disabled  FdbkBlocksVariant=Forward  IdealPFdbkVariant=Disabled  SatFdbkVariant=Disabled  DerivativeFilterVariant=Disabled  NVariant=Disabled  NCopyVariant=Disabled_SignalSpec  FilterICVariant=Disabled  IntegratorICVariant=InternalICs  ExternalResetVariant=Disabled  TRSumVariant=Passthrough  SumFdbkVariant=Disabled  SumVariant=Sum_PI  TsampFilterVariant=InternalTs  TsampNgainVariant=Passthrough  TsampIntegralVariant=Passthrough  ExternalSaturationOutDataTypeStr=Inherit: Same as second input
  Dq : Gain  Gain=Dq
  Product : Product
  Sum3 : Sum  Inputs=|-+
  Sum4 : Sum  Inputs=|++
  Sum5 : Sum  Inputs=|-+
  Sum6 : Sum  Inputs=|-+
  Is_d_ref : Outport
  Is_q_ref : Outport  Port=2
  wires:
  Sum5/1 -> Dq/1
  Sum3/1 -> Sum4/1
  Sum6/1 -> Discrete PID Controller/1
  Sum4/1 -> Discrete PID Controller3/1
  Vdc/1 -> Sum6/2
  Product/1 -> Sum4/2
  Dq/1 -> Product/1
  Qout/1 -> Sum3/2
  Activation signal/1 -> Product/2
  Vdc_ref/1 -> Sum6/1
  Discrete PID Controller3/1 -> Is_q_ref/1
  Qout_ref/1 -> Sum3/1
  Vpcc_rms_ref/1 -> Sum5/1
  Vpcc_rms/1 -> Sum5/2
  Discrete PID Controller/1 -> Is_d_ref/1

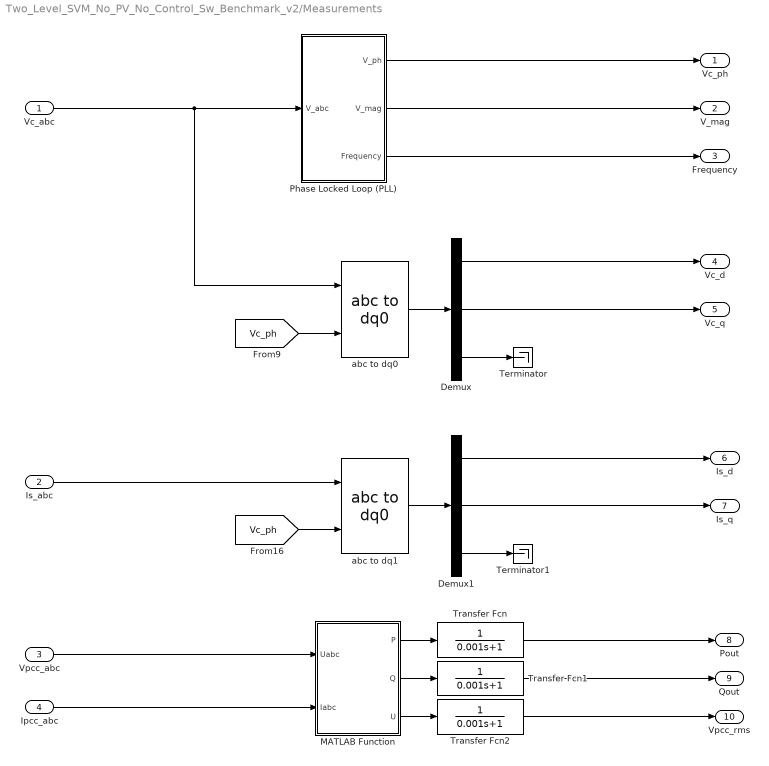
== system Two_Level_SVM_No_PV_No_Control_Sw_Benchmark_v2/Measurements ==
  Vc_abc : Inport
  Is_abc : Inport  Port=2
  Vpcc_abc : Inport  Port=3
  Ipcc_abc : Inport  Port=4
  Demux : Demux  Outputs=3
  Demux1 : Demux  Outputs=3
  MATLAB Function : MATLAB Function  TreatAsAtomicUnit=on
  Phase Locked Loop (PLL) : Subsystem
  Terminator : Terminator
  Terminator1 : Terminator
  Transfer Fcn : TransferFcn  Denominator=[0.001 1]
  Transfer Fcn1 : TransferFcn  Denominator=[0.001 1]
  Transfer Fcn2 : TransferFcn  Denominator=[0.001 1]
  abc to dq0 : spsabctodq0Lib/abc to dq0  Alignment=Aligned with phase A axis
  abc to dq1 : spsabctodq0Lib/abc to dq0  Alignment=Aligned with phase A axis
  Vc_ph : Outport
  V_mag : Outport  Port=2
  Frequency : Outport  Port=3
  Vc_d : Outport  Port=4
  Vc_q : Outport  Port=5
  Is_d : Outport  Port=6
  Is_q : Outport  Port=7
  Pout : Outport  Port=8
  Qout : Outport  Port=9
  Vpcc_rms : Outport  Port=10
  wires:
  Demux1/2 -> Is_q/1
  MATLAB Function/3(U) -> Transfer Fcn2/1
  Demux1/3 -> Terminator1/1
  [Vc_ph] -> abc to dq0/2
  [Vc_ph] -> abc to dq1/2
  Transfer Fcn1/1 -> Qout/1
  MATLAB Function/1(P) -> Transfer Fcn/1
  Transfer Fcn/1 -> Pout/1
  Vc_abc/1 -> abc to dq0/1, Phase Locked Loop (PLL)/1(V_abc)
  abc to dq1/1 -> Demux1/1
  abc to dq0/1 -> Demux/1
  Demux/3 -> Terminator/1
  Ipcc_abc/1 -> MATLAB Function/2(Iabc)
  MATLAB Function/2(Q) -> Transfer Fcn1/1
  Demux/1 -> Vc_d/1
  Transfer Fcn2/1 -> Vpcc_rms/1
  Demux1/1 -> Is_d/1
  Phase Locked Loop (PLL)/1(V_ph) -> Vc_ph/1
  Phase Locked Loop (PLL)/3(Frequency) -> Frequency/1
  Demux/2 -> Vc_q/1
  Phase Locked Loop (PLL)/2(V_mag) -> V_mag/1
  Is_abc/1 -> abc to dq1/1
  Vpcc_abc/1 -> MATLAB Function/1(Uabc)

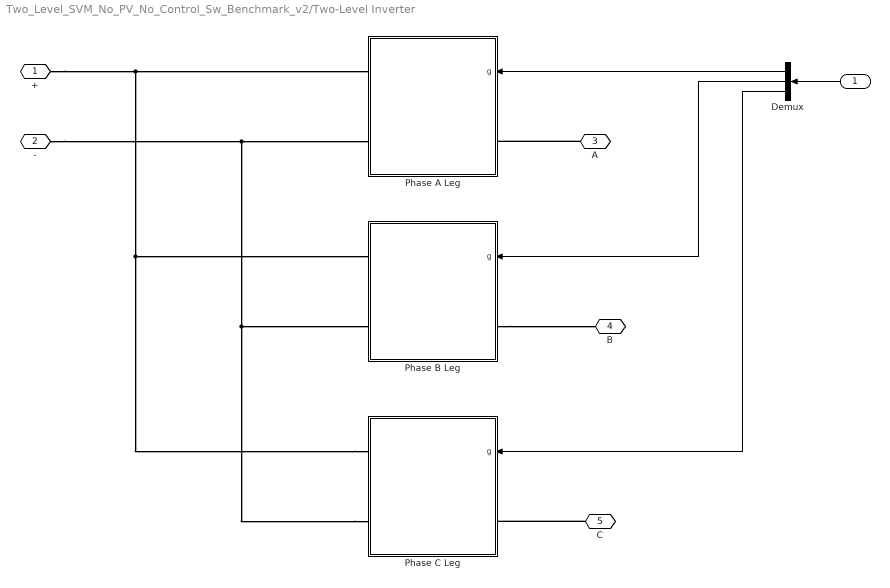
== system Two_Level_SVM_No_PV_No_Control_Sw_Benchmark_v2/Two-Level Inverter ==
  "  " : Inport
  Demux : Demux  Outputs=3
  Phase A Leg : Subsystem
      settings: PortSchema="{\"entries\":[{\"content\":{\"sides\":[{\"content\":{\"connectorIds\":[\"LConn1\",\"LConn2\"]},\"type\":\"ConnectorPlacement.EquallySpacedRectSide\",\"uuid\":\"85528a75-2624-46cc-84e7-425c3cd4a805\"},{\"content\":{\"connectorIds\":[\"In1\",\"RConn1\"],\"side\":\"RIGHT\"},\"type\":\"ConnectorPlacement.EquallySpacedRectSide\",\"uuid\":\"7112d789-799f-4f91-bfeb-6284407eaa2e\"},{\"content\":{\"connectorIds\":[],\"side\":\"TOP\"},\"type\":\"ConnectorPlacement.EquallySpacedRectSide\",\"uuid\":\"285c1ec0-b91b-4727-a014-0ce73a6f1ef0\"}]},\"type\":\"ConnectorPlacement.EquallySpacedConnector\",\"uuid\":\"0a31df6b-112a-4f38-954f-a98101aa9e43\"}],\"packageUris\":[\"http://schema.mathworks.com/mf0/Connector/R2020b\"],\"version\":\"1.0\"}"
  Phase B Leg : Subsystem
      settings: PortSchema="{\"entries\":[{\"content\":{\"sides\":[{\"content\":{\"connectorIds\":[\"LConn1\",\"LConn2\"]},\"type\":\"ConnectorPlacement.EquallySpacedRectSide\",\"uuid\":\"85528a75-2624-46cc-84e7-425c3cd4a805\"},{\"content\":{\"connectorIds\":[\"In1\",\"RConn1\"],\"side\":\"RIGHT\"},\"type\":\"ConnectorPlacement.EquallySpacedRectSide\",\"uuid\":\"7112d789-799f-4f91-bfeb-6284407eaa2e\"},{\"content\":{\"connectorIds\":[],\"side\":\"TOP\"},\"type\":\"ConnectorPlacement.EquallySpacedRectSide\",\"uuid\":\"285c1ec0-b91b-4727-a014-0ce73a6f1ef0\"}]},\"type\":\"ConnectorPlacement.EquallySpacedConnector\",\"uuid\":\"0a31df6b-112a-4f38-954f-a98101aa9e43\"}],\"packageUris\":[\"http://schema.mathworks.com/mf0/Connector/R2020b\"],\"version\":\"1.0\"}"
  Phase C Leg : Subsystem
      settings: PortSchema="{\"entries\":[{\"content\":{\"sides\":[{\"content\":{\"connectorIds\":[\"LConn1\",\"LConn2\"]},\"type\":\"ConnectorPlacement.EquallySpacedRectSide\",\"uuid\":\"85528a75-2624-46cc-84e7-425c3cd4a805\"},{\"content\":{\"connectorIds\":[\"In1\",\"RConn1\"],\"side\":\"RIGHT\"},\"type\":\"ConnectorPlacement.EquallySpacedRectSide\",\"uuid\":\"7112d789-799f-4f91-bfeb-6284407eaa2e\"},{\"content\":{\"connectorIds\":[],\"side\":\"TOP\"},\"type\":\"ConnectorPlacement.EquallySpacedRectSide\",\"uuid\":\"285c1ec0-b91b-4727-a014-0ce73a6f1ef0\"}]},\"type\":\"ConnectorPlacement.EquallySpacedConnector\",\"uuid\":\"0a31df6b-112a-4f38-954f-a98101aa9e43\"}],\"packageUris\":[\"http://schema.mathworks.com/mf0/Connector/R2020b\"],\"version\":\"1.0\"}"
  + : PMIOPort  Side=Right
  - : PMIOPort  Port=2  Side=Right
  A : PMIOPort  Port=3  Side=Left
  B : PMIOPort  Port=4  Side=Left
  C : PMIOPort  Port=5  Side=Left
  wires:
  "  "/1 -> Demux/1
  Demux/1 -> Phase A Leg/1(g)
  Demux/2 -> Phase B Leg/1(g)
  Demux/3 -> Phase C Leg/1(g)
  connections:
  A/RConn1 -- Phase A Leg/RConn1
  Phase B Leg/RConn1 -- B/RConn1
  C/RConn1 -- Phase C Leg/RConn1
  Phase C Leg/LConn1 -- Phase B Leg/LConn1 -- +/RConn1 -- Phase A Leg/LConn1
  Phase C Leg/LConn2 -- Phase B Leg/LConn2 -- -/RConn1 -- Phase A Leg/LConn2

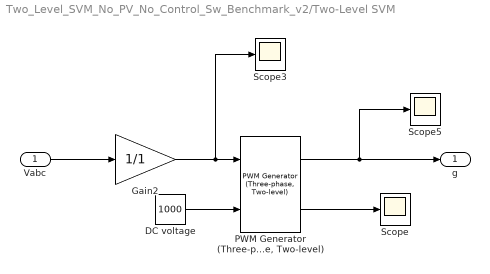
== system Two_Level_SVM_No_PV_No_Control_Sw_Benchmark_v2/Two-Level SVM ==
  Vabc : Inport
  DC voltage : Constant  Value=1000
  Gain2 : Gain  Gain=1/1
  "PWM Generator (Three-phase, Two-level)" : eePwmGeneratorTwoLevel/PWM Generator (Three-phase, Two-level)  PWMMode=Continuous PWM (CPWM)  CPWMMode=SVM: space vector modulation  DPWMMode=60 DPWM: 60 degree discontinuous PWM  fsw=fsw  Ts=1e-7
  Scope : Scope
  Scope3 : Scope
  Scope5 : Scope
  g : Outport
  wires:
  "PWM Generator (Three-phase, Two-level)"/1 -> g/1, Scope5/1
  Gain2/1 -> Scope3/1, "PWM Generator (Three-phase, Two-level)"/1
  "PWM Generator (Three-phase, Two-level)"/2 -> Scope/1
  DC voltage/1 -> "PWM Generator (Three-phase, Two-level)"/2
  Vabc/1 -> Gain2/1

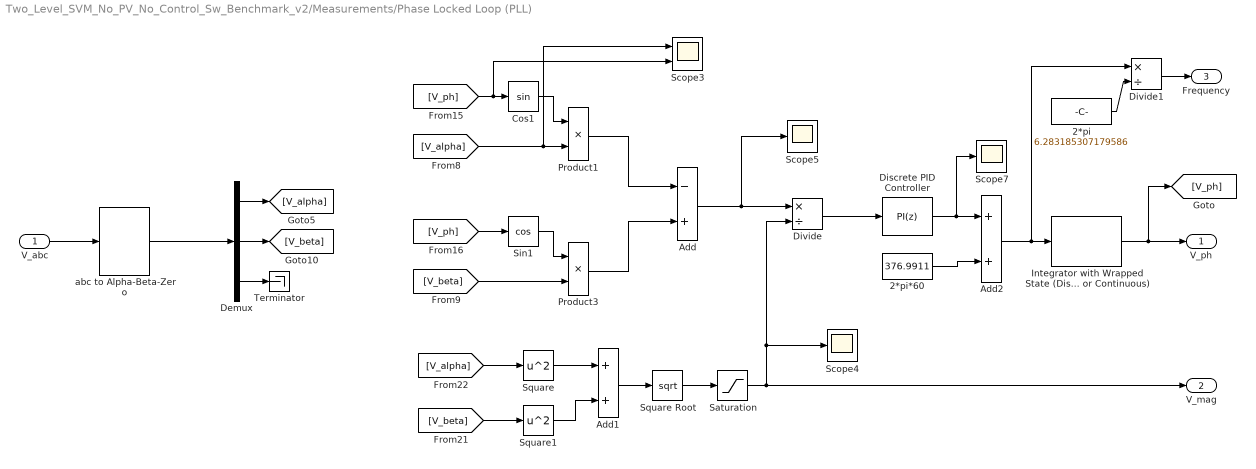
== system Two_Level_SVM_No_PV_No_Control_Sw_Benchmark_v2/Measurements/Phase Locked Loop (PLL) ==
  V_abc : Inport
  2*pi : Constant  Value=6.283185307179586
  2*pi*60 : Constant  Value=376.9911
  Add : Sum  Inputs=-+
  Add1 : Sum
  Add2 : Sum
  Cos1 : Trigonometry
  Demux : Demux  Outputs=3
  Discrete PID Controller : slpidlib/PID Controller  Controller=PI  Form=Parallel  TimeDomain=Discrete-time  UseExternalTs=off  SampleTime=-1  IntegratorMethod=Forward Euler  FilterMethod=Forward Euler  ControllerParametersSource=internal  P=Kp_PLL  I=Ki_PLL  UseKiTs=off  D=0  N=100  UseFilter=on  TunerSelectOption=Transfer Function Based (PID Tuner App)  InitialConditionSource=internal  InitialConditionForIntegrator=0  InitialConditionForFilter=0  DifferentiatorICPrevScaledInput=0  ExternalReset=none  TrackingMode=off  Kt=1  LimitOutput=off  SatLimitsSource=internal  UpperSaturationLimit=inf  LowerSaturationLimit=-inf  LinearizeAsGain=off  AntiWindupMode=none  Kb=1  LimitIntegrator=off  UpperIntegratorSaturationLimit=inf  LowerIntegratorSaturationLimit=-inf  POutMin=[]  POutMax=[]  IOutMin=[]  IOutMax=[]  DOutMin=[]  DOutMax=[]  NOutMin=[]  NOutMax=[]  SumOutMin=[]  SumOutMax=[]  SaturationOutMin=[]  SaturationOutMax=[]  PParamMin=[]  PParamMax=[]  IParamMin=[]  IParamMax=[]  DParamMin=[]  DParamMax=[]  NParamMin=[]  NParamMax=[]  KbParamMin=[]  KbParamMax=[]  KtParamMin=[]  KtParamMax=[]  KbOutMin=[]  KbOutMax=[]  KtOutMin=[]  KtOutMax=[]  IntegratorOutMin=[]  IntegratorOutMax=[]  FilterOutMin=[]  FilterOutMax=[]  SumI1OutMin=[]  SumI1OutMax=[]  SumI2OutMin=[]  SumI2OutMax=[]  SumI3OutMin=[]  SumI3OutMax=[]  SumI4OutMin=[]  SumI4OutMax=[]  SumDOutMin=[]  SumDOutMax=[]  DifferentiatorOutMin=[]  DifferentiatorOutMax=[]  FilterDiffOutCoefMin=[]  FilterDiffOutCoefMax=[]  ReciprocalOutMin=[]  ReciprocalOutMax=[]  SumDenOutMin=[]  SumDenOutMax=[]  SumNumOutMin=[]  SumNumOutMax=[]  DivideOutMin=[]  DivideOutMax=[]  UdiffTsProdOutMin=[]  UdiffTsProdOutMax=[]  NTsProdOutMin=[]  NTsProdOutMax=[]  UintegralTsProdOutMin=[]  UintegralTsProdOutMax=[]  UngainTsProdOutMin=[]  UngainTsProdOutMax=[]  ClampingZeroOutDataTypeStr=Inherit: Inherit via back propagation  ClampingZeroOutMin=[]  ClampingZeroOutMax=[]  FilterDenConstantOutDataTypeStr=Inherit: Inherit via back propagation  FilterDenConstantOutMin=[]  FilterDenConstantOutMax=[]  PCopyOutDataTypeStr=Inherit: Inherit via back propagation  PCopyOutMin=[]  PCopyOutMax=[]  NCopyOutDataTypeStr=Inherit: Inherit via back propagation  NCopyOutMin=[]  NCopyOutMax=[]  IntegratorContinuousStateAttributes=''  IntegratorStateMustResolveToSignalObject=off  IntegratorRTWStateStorageClass=Auto  FilterContinuousStateAttributes=''  FilterStateMustResolveToSignalObject=off  FilterRTWStateStorageClass=Auto  ParallelPVariant=InternalParameters  IdealPVariant=Disabled  IVariant=InternalParameters  DVariant=Disabled  IntegratorVariant=Discrete  SatVariant=Disabled  AWVariant=Passthrough  PCopyVariant=Disabled  TRVariant=Disabled  FdbkBlocksVariant=Forward  IdealPFdbkVariant=Disabled  SatFdbkVariant=Disabled  DerivativeFilterVariant=Disabled  NVariant=Disabled  NCopyVariant=Disabled_SignalSpec  FilterICVariant=Disabled  IntegratorICVariant=InternalICs  ExternalResetVariant=Disabled  TRSumVariant=Passthrough  SumFdbkVariant=Disabled  SumVariant=Sum_PI  TsampFilterVariant=InternalTs  TsampNgainVariant=Passthrough  TsampIntegralVariant=Passthrough  ExternalSaturationOutDataTypeStr=Inherit: Same as second input
  Divide : Product  Inputs=*/
  Divide1 : Product  Inputs=*/
  Integrator with Wrapped State (Discrete or Continuous) : eeGeneralControl/Integrator with Wrapped State (Discrete or Continuous)  LabelModeActiveChoice=Discrete  WrappedStateUpperValue=pi  WrappedStateLowerValue=-pi  x0=0  Ts=-1
  Product1 : Product
  Product3 : Product
  Saturation : Saturate  UpperLimit=inf  LowerLimit=0.001
  Scope3 : Scope  NumInputPorts=2
  Scope4 : Scope
  Scope5 : Scope
  Scope7 : Scope
  Sin1 : Trigonometry  Operator=cos
  Square : Math  Operator=square
  Square Root : Sqrt
  Square1 : Math  Operator=square
  Terminator : Terminator
  abc to Alpha-Beta-Zero : spsabctoAlphaBetaZeroLib/abc to Alpha-Beta-Zero
  V_ph : Outport
  V_mag : Outport  Port=2
  Frequency : Outport  Port=3
  wires:
  Saturation/1 -> V_mag/1, Scope4/1, Divide/2
  [V_alpha] -> Square/1
  Discrete PID Controller/1 -> Scope7/1, Add2/1
  Cos1/1 -> Product1/1
  abc to Alpha-Beta-Zero/1 -> Demux/1
  Demux/1 -> [V_alpha]
  [V_alpha] -> Scope3/1, Product1/2
  Square/1 -> Add1/1
  Demux/2 -> [V_beta]
  V_abc/1 -> abc to Alpha-Beta-Zero/1
  Product3/1 -> Add/2
  [V_ph] -> Scope3/2, Cos1/1
  [V_beta] -> Product3/2
  Add2/1 -> Divide1/1, Integrator with Wrapped State (Discrete or Continuous)/1
  Square1/1 -> Add1/2
  [V_ph] -> Sin1/1
  Demux/3 -> Terminator/1
  Product1/1 -> Add/1
  Add/1 -> Scope5/1, Divide/1
  Sin1/1 -> Product3/1
  2*pi*60/1 -> Add2/2
  Add1/1 -> Square Root/1
  Square Root/1 -> Saturation/1
  [V_beta] -> Square1/1
  Divide/1 -> Discrete PID Controller/1
  Integrator with Wrapped State (Discrete or Continuous)/1 -> [V_ph], V_ph/1
  Divide1/1 -> Frequency/1
  2*pi/1 -> Divide1/2

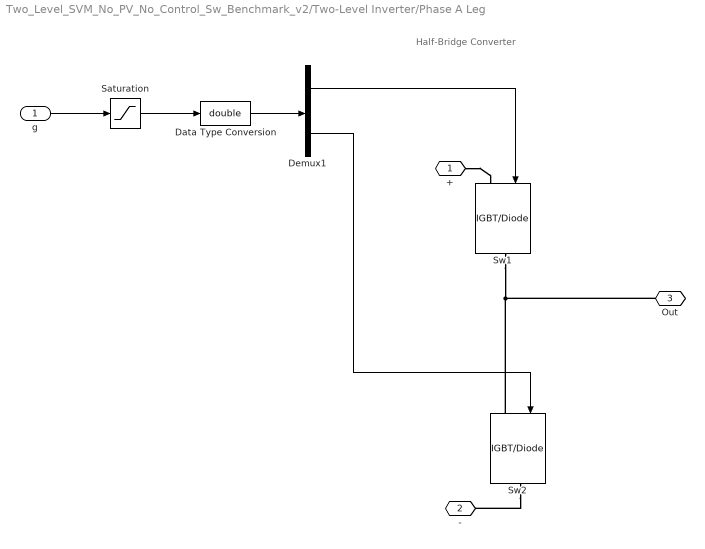
== system Two_Level_SVM_No_PV_No_Control_Sw_Benchmark_v2/Two-Level Inverter/Phase A Leg ==
  note: Half-Bridge Converter
  g : Inport
  Data Type Conversion : DataTypeConversion  OutDataTypeStr=double  SaturateOnIntegerOverflow=off  RndMeth=Floor
  Demux1 : Demux  Outputs=2
  Saturation : Saturate  UpperLimit=1  LowerLimit=0
  Sw1 : spsIGBTDiodeLib/IGBT//Diode  Ron=Ron  Rs=Rs  Cs=Cs  Measurements=off
  Sw2 : spsIGBTDiodeLib/IGBT//Diode  Ron=Ron  Rs=Rs  Cs=Cs  Measurements=off
  + : PMIOPort  Side=Left
  - : PMIOPort  Port=2  Side=Left
  Out : PMIOPort  Port=3  Side=Right
  wires:
  Data Type Conversion/1 -> Demux1/1
  Demux1/1 -> Sw1/1
  Demux1/2 -> Sw2/1
  Saturation/1 -> Data Type Conversion/1
  g/1 -> Saturation/1
  connections:
  +/RConn1 -- Sw1/LConn1
  Sw1/RConn1 -- Out/RConn1 -- Sw2/LConn1
  Sw2/RConn1 -- -/RConn1

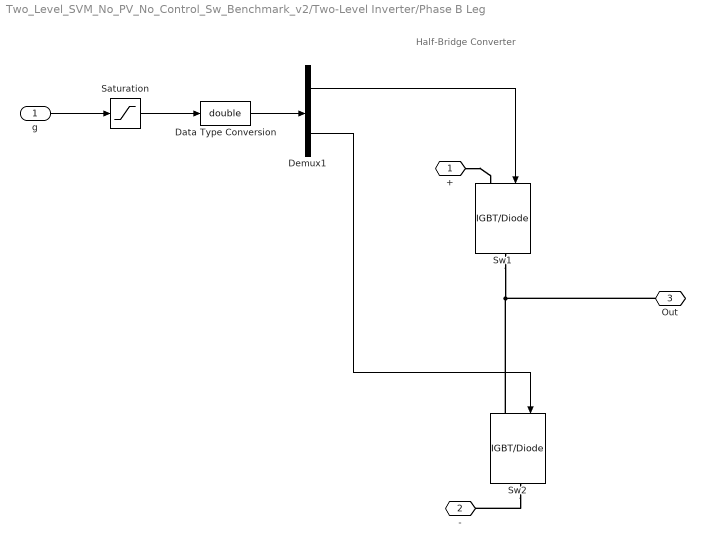
== system Two_Level_SVM_No_PV_No_Control_Sw_Benchmark_v2/Two-Level Inverter/Phase B Leg ==
  note: Half-Bridge Converter
  g : Inport
  Data Type Conversion : DataTypeConversion  OutDataTypeStr=double  SaturateOnIntegerOverflow=off  RndMeth=Floor
  Demux1 : Demux  Outputs=2
  Saturation : Saturate  UpperLimit=1  LowerLimit=0
  Sw1 : spsIGBTDiodeLib/IGBT//Diode  Ron=Ron  Rs=Rs  Cs=Cs  Measurements=off
  Sw2 : spsIGBTDiodeLib/IGBT//Diode  Ron=Ron  Rs=Rs  Cs=Cs  Measurements=off
  + : PMIOPort  Side=Left
  - : PMIOPort  Port=2  Side=Left
  Out : PMIOPort  Port=3  Side=Right
  wires:
  Data Type Conversion/1 -> Demux1/1
  Demux1/1 -> Sw1/1
  Demux1/2 -> Sw2/1
  Saturation/1 -> Data Type Conversion/1
  g/1 -> Saturation/1
  connections:
  +/RConn1 -- Sw1/LConn1
  Sw2/LConn1 -- Sw1/RConn1 -- Out/RConn1
  Sw2/RConn1 -- -/RConn1

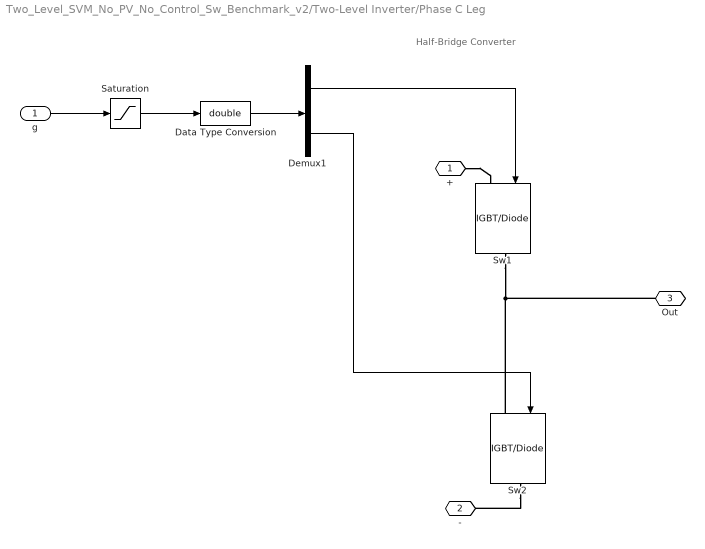
== system Two_Level_SVM_No_PV_No_Control_Sw_Benchmark_v2/Two-Level Inverter/Phase C Leg ==
  note: Half-Bridge Converter
  g : Inport
  Data Type Conversion : DataTypeConversion  OutDataTypeStr=double  SaturateOnIntegerOverflow=off  RndMeth=Floor
  Demux1 : Demux  Outputs=2
  Saturation : Saturate  UpperLimit=1  LowerLimit=0
  Sw1 : spsIGBTDiodeLib/IGBT//Diode  Ron=Ron  Rs=Rs  Cs=Cs  Measurements=off
  Sw2 : spsIGBTDiodeLib/IGBT//Diode  Ron=Ron  Rs=Rs  Cs=Cs  Measurements=off
  + : PMIOPort  Side=Left
  - : PMIOPort  Port=2  Side=Left
  Out : PMIOPort  Port=3  Side=Right
  wires:
  Data Type Conversion/1 -> Demux1/1
  Demux1/1 -> Sw1/1
  Demux1/2 -> Sw2/1
  Saturation/1 -> Data Type Conversion/1
  g/1 -> Saturation/1
  connections:
  +/RConn1 -- Sw1/LConn1
  Sw2/LConn1 -- Sw1/RConn1 -- Out/RConn1
  Sw2/RConn1 -- -/RConn1
